simulink library "halin"  (R2021b)
settings: Solver=VariableStepAuto  StartTime=0.0  StopTime=10.0  RelTol=1e-3
undefined symbols (not defined in the file): TRUE
libraries: FVT_lib x37, hcu_lib x31
(part 4 of 4)

== system halin/HAL_IN/CAN4/ZRR_CE100_1/ZRRBCMPLampSta ==
  ZRR_BCM_PLamp_Sta : Inport
  UnitConverter : DataTypeConversion  OutDataTypeStr=uint8
  VHAL_ZRRBCMPLampSta_flg : Outport
  wires:
  UnitConverter/1 -> VHAL_ZRRBCMPLampSta_flg/1
  ZRR_BCM_PLamp_Sta/1 -> UnitConverter/1

== system halin/HAL_IN/CAN4/ZRR_CE100_1/ZRRBCMRRTurnLpCSta ==
  ZRR_BCM_RRTurnLpC_Sta : Inport
  UnitConverter : DataTypeConversion  OutDataTypeStr=uint8
  convert_in : FVT_lib/hal/convert_in  gain=0.025  offset=0
  VHAL_ZRRBCMRRTurnLpCSta_A : Outport
  wires:
  convert_in/1 -> VHAL_ZRRBCMRRTurnLpCSta_A/1
  UnitConverter/1 -> convert_in/1
  ZRR_BCM_RRTurnLpC_Sta/1 -> UnitConverter/1

== system halin/HAL_IN/CAN4/ZRR_CE100_1/ZRRBCMSTOPSW2Sta ==
  ZRR_BCM_STOPSW2_Sta : Inport
  UnitConverter : DataTypeConversion  OutDataTypeStr=uint8
  VHAL_ZRRBCMSTOPSW2Sta_flg : Outport
  wires:
  UnitConverter/1 -> VHAL_ZRRBCMSTOPSW2Sta_flg/1
  ZRR_BCM_STOPSW2_Sta/1 -> UnitConverter/1

== system halin/HAL_IN/CAN4/ZRR_CE100_1/ZRRBCMSTOPSWSta ==
  ZRR_BCM_STOPSW_Sta : Inport
  UnitConverter : DataTypeConversion  OutDataTypeStr=uint8
  VHAL_ZRRBCMSTOPSWSta_flg : Outport
  wires:
  UnitConverter/1 -> VHAL_ZRRBCMSTOPSWSta_flg/1
  ZRR_BCM_STOPSW_Sta/1 -> UnitConverter/1

== system halin/HAL_IN/CAN4/zGW_CANRr1_C50_0/DCDCEnSta ==
  DCDC_En_Sta : Inport
  UnitConverter : DataTypeConversion  OutDataTypeStr=uint8
  VHAL_DCDCEnSta_enum : Outport
  wires:
  UnitConverter/1 -> VHAL_DCDCEnSta_enum/1
  DCDC_En_Sta/1 -> UnitConverter/1

== system halin/HAL_IN/CAN4/zGW_CANRr1_C50_0/DCDCErrLvSta ==
  DCDC_ErrLv_Sta : Inport
  UnitConverter : DataTypeConversion  OutDataTypeStr=uint8
  VHAL_DCDCErrLvSta_enum : Outport
  wires:
  UnitConverter/1 -> VHAL_DCDCErrLvSta_enum/1
  DCDC_ErrLv_Sta/1 -> UnitConverter/1

== system halin/HAL_IN/CAN4/zGW_CANRr1_C50_0/DCDCOutVolSta ==
  DCDC_OutVol_Sta : Inport
  UnitConverter : DataTypeConversion  OutDataTypeStr=uint16
  convert_in : FVT_lib/hal/convert_in  gain=0.1  offset=0
  VHAL_DCDCOutVolSta_V : Outport
  wires:
  convert_in/1 -> VHAL_DCDCOutVolSta_V/1
  UnitConverter/1 -> convert_in/1
  DCDC_OutVol_Sta/1 -> UnitConverter/1

== system halin/HAL_IN/CAN4/zGW_CANRr1_C50_0/DCDCTempSta ==
  DCDC_Temp_Sta : Inport
  UnitConverter : DataTypeConversion  OutDataTypeStr=uint8
  convert_in : FVT_lib/hal/convert_in  gain=1  offset=-40
  VHAL_DCDCTempSta_C : Outport
  wires:
  convert_in/1 -> VHAL_DCDCTempSta_C/1
  UnitConverter/1 -> convert_in/1
  DCDC_Temp_Sta/1 -> UnitConverter/1

== system halin/HAL_IN/CAN4/zGW_CANRr1_C50_0/EACEnSta ==
  EAC_En_Sta : Inport
  UnitConverter : DataTypeConversion  OutDataTypeStr=uint8
  VHAL_EACEnSta_enum : Outport
  wires:
  UnitConverter/1 -> VHAL_EACEnSta_enum/1
  EAC_En_Sta/1 -> UnitConverter/1

== system halin/HAL_IN/CAN4/zGW_CANRr1_C50_0/EACErrLvSta ==
  EAC_ErrLv_Sta : Inport
  UnitConverter : DataTypeConversion  OutDataTypeStr=uint8
  VHAL_EACErrLvSta_enum : Outport
  wires:
  UnitConverter/1 -> VHAL_EACErrLvSta_enum/1
  EAC_ErrLv_Sta/1 -> UnitConverter/1

== system halin/HAL_IN/CAN4/zGW_CANRr1_C50_0/EACInvTempSta ==
  EAC_InvTemp_Sta : Inport
  UnitConverter : DataTypeConversion  OutDataTypeStr=uint8
  convert_in : FVT_lib/hal/convert_in  gain=1  offset=-40
  VHAL_EACInvTempSta_C : Outport
  wires:
  convert_in/1 -> VHAL_EACInvTempSta_C/1
  UnitConverter/1 -> convert_in/1
  EAC_InvTemp_Sta/1 -> UnitConverter/1

== system halin/HAL_IN/CAN4/zGW_CANRr1_C50_0/EHPSEnSta ==
  EHPS_En_Sta : Inport
  UnitConverter : DataTypeConversion  OutDataTypeStr=uint8
  VHAL_EHPSEnSta_enum : Outport
  wires:
  UnitConverter/1 -> VHAL_EHPSEnSta_enum/1
  EHPS_En_Sta/1 -> UnitConverter/1

== system halin/HAL_IN/CAN4/zGW_CANRr1_C50_0/EHPSErrLvSta ==
  EHPS_ErrLv_Sta : Inport
  UnitConverter : DataTypeConversion  OutDataTypeStr=uint8
  VHAL_EHPSErrLvSta_enum : Outport
  wires:
  UnitConverter/1 -> VHAL_EHPSErrLvSta_enum/1
  EHPS_ErrLv_Sta/1 -> UnitConverter/1

== system halin/HAL_IN/CAN4/zGW_CANRr1_C50_0/EHPSInvTempSta ==
  EHPS_InvTemp_Sta : Inport
  UnitConverter : DataTypeConversion  OutDataTypeStr=uint8
  convert_in : FVT_lib/hal/convert_in  gain=1  offset=-40
  VHAL_EHPSInvTempSta_C : Outport
  wires:
  convert_in/1 -> VHAL_EHPSInvTempSta_C/1
  UnitConverter/1 -> convert_in/1
  EHPS_InvTemp_Sta/1 -> UnitConverter/1

== system halin/HAL_IN/CAN4/zGW_CANRr1_C50_0/EHPSMotorSpdSta ==
  EHPS_MotorSpd_Sta : Inport
  UnitConverter : DataTypeConversion  OutDataTypeStr=uint16
  convert_in : FVT_lib/hal/convert_in  gain=0.5  offset=-5000
  VHAL_EHPSMotorSpdSta_rpm : Outport
  wires:
  convert_in/1 -> VHAL_EHPSMotorSpdSta_rpm/1
  UnitConverter/1 -> convert_in/1
  EHPS_MotorSpd_Sta/1 -> UnitConverter/1

== system halin/HAL_IN/CAN4/zGW_CANRr1_C50_0/PDUACRlySta ==
  PDU_ACRly_Sta : Inport
  UnitConverter : DataTypeConversion  OutDataTypeStr=uint8
  VHAL_PDUACRlySta_enum : Outport
  wires:
  UnitConverter/1 -> VHAL_PDUACRlySta_enum/1
  PDU_ACRly_Sta/1 -> UnitConverter/1

== system halin/HAL_IN/CAN4/zGW_CANRr1_C50_0/PDUDCDCEACEHPSHVLoopSta ==
  PDU_DCDCEACEHPSHVLoop_Sta : Inport
  UnitConverter : DataTypeConversion  OutDataTypeStr=uint8
  VHAL_PDUDCDCEACEHPSHVLoopSta_enum : Outport
  wires:
  UnitConverter/1 -> VHAL_PDUDCDCEACEHPSHVLoopSta_enum/1
  PDU_DCDCEACEHPSHVLoop_Sta/1 -> UnitConverter/1

== system halin/HAL_IN/CAN4/zGW_CANRr1_C50_0/PDUDCDCEACEHPSPreRlySta ==
  PDU_DCDCEACEHPSPreRly_Sta : Inport
  UnitConverter : DataTypeConversion  OutDataTypeStr=uint8
  VHAL_PDUDCDCEACEHPSPreRlySta_enum : Outport
  wires:
  UnitConverter/1 -> VHAL_PDUDCDCEACEHPSPreRlySta_enum/1
  PDU_DCDCEACEHPSPreRly_Sta/1 -> UnitConverter/1

== system halin/HAL_IN/CAN4/zGW_CANRr1_C50_0/PDUDCDCEACEHPSRlySta ==
  PDU_DCDCEACEHPSRly_Sta : Inport
  UnitConverter : DataTypeConversion  OutDataTypeStr=uint8
  VHAL_PDUDCDCEACEHPSRlySta_enum : Outport
  wires:
  UnitConverter/1 -> VHAL_PDUDCDCEACEHPSRlySta_enum/1
  PDU_DCDCEACEHPSRly_Sta/1 -> UnitConverter/1

== system halin/HAL_IN/CAN4/zGW_CANRr1_C50_0/PDUHVILSta ==
  PDU_HVIL_Sta : Inport
  UnitConverter : DataTypeConversion  OutDataTypeStr=uint8
  VHAL_PDUHVILSta_enum : Outport
  wires:
  UnitConverter/1 -> VHAL_PDUHVILSta_enum/1
  PDU_HVIL_Sta/1 -> UnitConverter/1

== system halin/HAL_IN/CAN4/zGW_CANRr1_C50_0/PDUMCUHVLoopSta ==
  PDU_MCUHVLoop_Sta : Inport
  UnitConverter : DataTypeConversion  OutDataTypeStr=uint8
  VHAL_PDUMCUHVLoopSta_enum : Outport
  wires:
  UnitConverter/1 -> VHAL_PDUMCUHVLoopSta_enum/1
  PDU_MCUHVLoop_Sta/1 -> UnitConverter/1

== system halin/HAL_IN/CAN4/zGW_CANRr1_C50_0/PDUMCUPosRlySta ==
  PDU_MCUPosRly_Sta : Inport
  UnitConverter : DataTypeConversion  OutDataTypeStr=uint8
  VHAL_PDUMCUPosRlySta_enum : Outport
  wires:
  UnitConverter/1 -> VHAL_PDUMCUPosRlySta_enum/1
  PDU_MCUPosRly_Sta/1 -> UnitConverter/1

== system halin/HAL_IN/CAN4/zGW_CANRr1_C50_0/PDUMCUPreRlySta ==
  PDU_MCUPreRly_Sta : Inport
  UnitConverter : DataTypeConversion  OutDataTypeStr=uint8
  VHAL_PDUMCUPreRlySta_enum : Outport
  wires:
  UnitConverter/1 -> VHAL_PDUMCUPreRlySta_enum/1
  PDU_MCUPreRly_Sta/1 -> UnitConverter/1

== system halin/HAL_IN/CAN4/zGW_CANRr1_C50_0/PDUSelfChkSta ==
  PDU_SelfChk_Sta : Inport
  UnitConverter : DataTypeConversion  OutDataTypeStr=uint8
  VHAL_PDUSelfChkSta_enum : Outport
  wires:
  UnitConverter/1 -> VHAL_PDUSelfChkSta_enum/1
  PDU_SelfChk_Sta/1 -> UnitConverter/1
